simulink model "Model_1_1"  (R2024a)
settings: Solver=ode15s  StartTime=0.0  StopTime=100  FixedStep=0.0001  MaxStep=0.01  RelTol=1e-3  AbsTol=1e-3  EnableMultiTasking=on
model workspace (MATLAB code in the model file):
  | F_load_x= 2e3; %[N]
  | F_load_y= 1e4; %[N]
  | 
  | d=0.01;   %[m]
  | l=1;      %[m]
  | L=l;      %[m] Node distance
  | H=L*cos(pi/6); %[m] Node distance
  | Density=7800; %[kg/m^3]
  | E=210;   %[GPa]
  | G=79;    %[GPa]
  | bm=0.01; %[1/s] Default
  | bk=0.01; %[s] Default
  | 
  | b_rj=1; %[N*m*s/rad] Damp.Coef.Revolut joints
  | 
  | Size_frame=30; %[pixel]
undefined symbols (not defined in the file): F_x, F_y, X, Y, Z
libraries: sm_lib x58, nesl_utility x15, fl_lib x6, simulink x1
(part 1 of 2)
settings Model: NumberOfSteps=100000  Creator=Ing. Štefan Ondočko  LastModifiedBy=Ing. Štefan Ondočko
settings SolverCC: AutoScaleAbsTol=off  MaxZcPerStep=1
settings DataIOCC: LimitDataPoints=on  MaxDataPoints=10000  ReturnWorkspaceOutputs=off
settings OptimizationCC: ReuseModelBlockBuffer=off  LifeSpan=inf
settings DebuggingCC: UnconnectedInputMsg=warning  UnconnectedOutputMsg=warning  UnconnectedLineMsg=warning  AllowSymbolicDim=off  SubsystemReferenceDiagnosticForUnitTest=warning  SFUnexpectedBacktrackingDiag=warning  SFNoUnconditionalDefaultTransitionDiag=warning  SFExecutionAtInitializationDiag=none  ArithmeticOperatorsInVariantConditions=warning
settings ModelReferenceCC: EnableRefExpFcnMdlSchedulingChecks=on
settings SFSimCC: SimUseLocalCustomCode=off  CustomCodeUndefinedFunction=UseInterfaceOnly
settings RTWCC: RTWUseLocalCustomCode=off  GPUComputeCapability=3.5  DLArmComputeVersion=19.05
settings CodeAppCC: StateflowObjectComments=on
settings GRTTargetCC: TargetLangStandard=C89/C90 (ANSI)
settings ConfigComp: CovMetricSettings=dw  CovSaveCumulativeToWorkspaceVar=on  CovSaveSingleToWorkspaceVar=on  CovExternalEMLEnable=off  CovSFcnEnable=off
settings SimscapeCC: SimscapeLogType=all  SimscapeLogSimulationStatistics=on  SimscapeLogDataHistory=10000
settings ExplorerConfigSet: InternalSimMechanicsExplorerSettings="<ExplorerConfiguration><canonicalview>default</canonicalview><AnimationSetting><BasePlaybackSpeed>1.0</BasePlaybackSpeed><PlaybackSpeedFactor>2.0</PlaybackSpeedFactor></AnimationSetting><TilePanel><TileInfo><Tiles Columns=\"1\" Count=\"1\" Rows=\"1\"><Column Weight=\"1\"/><Row Weight=\"1\"/><Tile Height=\"1\" Width=\"1\" X=\"0\" Y=\"0\"/></Tiles></TileInfo><SceneInfo><SceneViewer><BGColor><R>1</R><G>1</G><B>1</B></BGColor><Camera><DoPerspective>off</DoPerspective><Position><X>1.34160017439744395</X><Y>2.43472426416735921</Y><Z>3.19868175252832421</Z></Position><Center><X>1.34160017439744395</X><Y>2.43472426416735921</Y><Z>1.1802899990698279e-08</Z></Center><Up><X>0</X><Y>1</Y><Z>-0</Z></Up><ViewLimDist>1</ViewLimDist><YLim>3.18022072065698147</YLim><XLim>1.97030216076793452</XLim></Camera></SceneViewer></SceneInfo></TilePanel><MechEditorPanel><Cameras/><GfxPanelCameraMap/><VideoCreator><PlaybackSpeedRatio>1.0</PlaybackSpeedRatio><FrameRate>30</FrameRate><VideoFormat>Motion JPEG AVI</VideoFormat><FrameSize>auto</FrameSize></VideoCreator></MechEditorPanel></ExplorerConfiguration>"

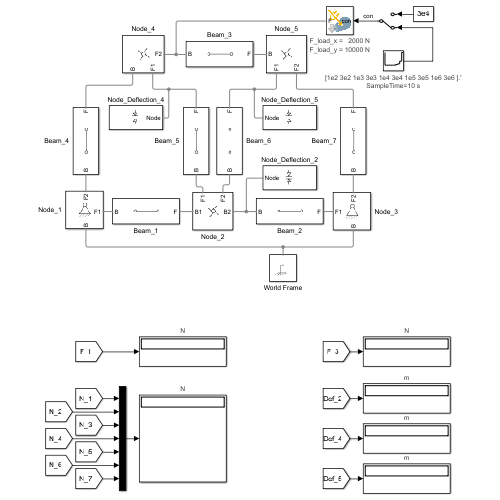
[thumbnail: Simulink's stored preview of the top-level diagram]
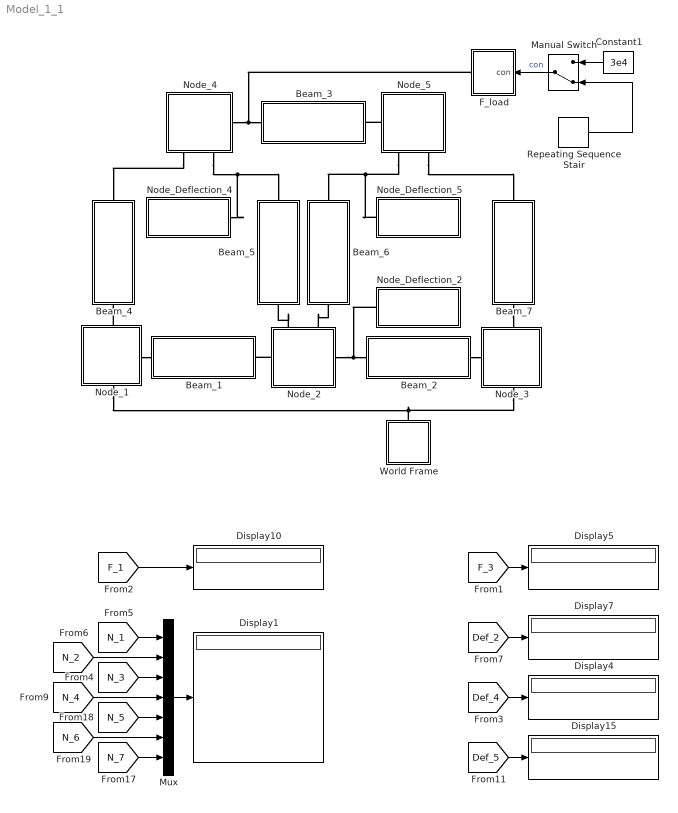
== system Model_1_1 ==
  Beam_1 : Subsystem
  Beam_2 : Subsystem
  Beam_3 : Subsystem
  Beam_4 : Subsystem
  Beam_5 : Subsystem
  Beam_6 : Subsystem
  Beam_7 : Subsystem
  Constant1 : Constant  Value=3e4
  Display{1,4..5,7,10,15} (6 alike) : Display
      Display1 settings: Description=N  AttributesFormatString=%<Description>  Format=long_e
      Display10 settings: Description=N  AttributesFormatString=%<Description>  Format=long_e
      Display15 settings: Description=m  AttributesFormatString=%<Description>  Format=long_e
      Display4 settings: Description=m  AttributesFormatString=%<Description>  Format=long_e
      Display5 settings: Description=N  AttributesFormatString=%<Description>  Format=long_e
      Display7 settings: Description=m  AttributesFormatString=%<Description>  Format=long_e
  F_load : Subsystem  mask{Fx=F_load_x, Fy=F_load_y, F=norm([F_x F_y])}
      mask prompts: Fx "Load Fx (N)"; Fy "Load Fy (N)"; F "Load F (N)"
      settings: AttributesFormatString=|
      | %<Fx> =   2000 N
      | %<Fy> = 10000 N
      mask Display: image('D:sila_F.png');
  Manual Switch : ManualSwitch  CurrentSetting=0
  Mux : Mux  Inputs=7
  Node_1 : Subsystem
      settings: PortSchema="{\"entries\":[{\"content\":{\"sides\":[{\"content\":{},\"type\":\"ConnectorPlacement.EquallySpacedRectSide\",\"uuid\":\"d437545a-b6cd-405c-92f5-dfd428dd316c\"},{\"content\":{\"connectorIds\":[\"RConn1\"],\"side\":\"RIGHT\"},\"type\":\"ConnectorPlacement.EquallySpacedRectSide\",\"uuid\":\"a6c866cb-015a-4ba6-a725-1ad5f0a48a96\"},{\"content\":{\"connectorIds\":[\"LConn1\"],\"side\":\"TOP\"},\"type\":\"ConnectorPlacement.EquallySpacedRectSide\",\"uuid\":\"8c34f49c-4b46-4dd5-857b-cc1f00e0721b\"},{\"content\":{\"connectorIds\":[\"RConn2\"],\"side\":\"BOTTOM\"},\"type\":\"ConnectorPlacement.EquallySpacedRectSide\",\"uuid\":\"e1836308-c472-4635-822e-d84e1319bcc1\"}]},\"type\":\"ConnectorPlacement.EquallySpacedConnector\",\"uuid\":\"28d0e514-5749-47ac-8c9d-469c58f8fea4\"}],\"packageUris\":[\"http://schema.mathworks.com/mf0/Connector/R2020b\"],\"version\":\"1.0\"}"
  Node_2 : Subsystem
      settings: PortSchema="{\"entries\":[{\"content\":{\"sides\":[{\"content\":{\"connectorIds\":[\"LConn1\"]},\"type\":\"ConnectorPlacement.EquallySpacedRectSide\",\"uuid\":\"afef6c51-8d1a-46bc-b1c6-0f4974bd4a7e\"},{\"content\":{\"connectorIds\":[\"RConn1\"],\"side\":\"RIGHT\"},\"type\":\"ConnectorPlacement.EquallySpacedRectSide\",\"uuid\":\"d0b349a1-0497-425d-af85-a98150ab0495\"},{\"content\":{\"side\":\"TOP\"},\"type\":\"ConnectorPlacement.EquallySpacedRectSide\",\"uuid\":\"d0ddbf7d-56c5-4c92-a64b-8a4c4ad659a6\"},{\"content\":{\"connectorIds\":[\"RConn2\",\"RConn3\"],\"side\":\"BOTTOM\"},\"type\":\"ConnectorPlacement.EquallySpacedRectSide\",\"uuid\":\"41f51937-efee-41b9-946e-3cb9cf7bb08c\"}]},\"type\":\"ConnectorPlacement.EquallySpacedConnector\",\"uuid\":\"81c85225-024f-4f40-8315-d14bb13695f6\"}],\"packageUris\":[\"http://schema.mathworks.com/mf0/Connector/R2020b\"],\"version\":\"1.0\"}"
  Node_3 : Subsystem
      settings: PortSchema="{\"entries\":[{\"content\":{\"sides\":[{\"content\":{\"connectorIds\":[\"LConn1\"]},\"type\":\"ConnectorPlacement.EquallySpacedRectSide\",\"uuid\":\"c52cac6f-2005-4bfe-89ae-e2a0406bbacd\"},{\"content\":{\"side\":\"RIGHT\"},\"type\":\"ConnectorPlacement.EquallySpacedRectSide\",\"uuid\":\"5ceadddb-1bc3-405b-9850-d33e8ff0b50d\"},{\"content\":{\"connectorIds\":[\"LConn2\"],\"side\":\"TOP\"},\"type\":\"ConnectorPlacement.EquallySpacedRectSide\",\"uuid\":\"947f3bae-c8fa-4b23-8ea1-709fee7d1677\"},{\"content\":{\"connectorIds\":[\"RConn1\"],\"side\":\"BOTTOM\"},\"type\":\"ConnectorPlacement.EquallySpacedRectSide\",\"uuid\":\"f9cd605e-29e4-49b7-a86d-9958a73b4d00\"}]},\"type\":\"ConnectorPlacement.EquallySpacedConnector\",\"uuid\":\"8856fa92-01df-438d-a79d-88950b3b721b\"}],\"packageUris\":[\"http://schema.mathworks.com/mf0/Connector/R2020b\"],\"version\":\"1.0\"}"
  Node_4 : Subsystem
      settings: PortSchema="{\"entries\":[{\"content\":{\"sides\":[{\"content\":{},\"type\":\"ConnectorPlacement.EquallySpacedRectSide\",\"uuid\":\"beaa1c3e-db26-40c7-ae29-b74306d70d13\"},{\"content\":{\"connectorIds\":[\"RConn1\"],\"side\":\"RIGHT\"},\"type\":\"ConnectorPlacement.EquallySpacedRectSide\",\"uuid\":\"a69b9587-50d9-4008-b2d1-888e5f048004\"},{\"content\":{\"connectorIds\":[\"LConn1\",\"LConn2\"],\"side\":\"TOP\"},\"type\":\"ConnectorPlacement.EquallySpacedRectSide\",\"uuid\":\"2aa7e189-65af-4eae-a330-225785720398\"}]},\"type\":\"ConnectorPlacement.EquallySpacedConnector\",\"uuid\":\"ac87f387-ad78-4612-b729-74bf7414ceb5\"}],\"packageUris\":[\"http://schema.mathworks.com/mf0/Connector/R2020b\"],\"version\":\"1.0\"}"
  Node_5 : Subsystem
      settings: PortSchema="{\"entries\":[{\"content\":{\"sides\":[{\"content\":{\"connectorIds\":[\"LConn1\"]},\"type\":\"ConnectorPlacement.EquallySpacedRectSide\",\"uuid\":\"beaa1c3e-db26-40c7-ae29-b74306d70d13\"},{\"content\":{\"side\":\"RIGHT\"},\"type\":\"ConnectorPlacement.EquallySpacedRectSide\",\"uuid\":\"a69b9587-50d9-4008-b2d1-888e5f048004\"},{\"content\":{\"connectorIds\":[\"LConn2\",\"LConn3\"],\"side\":\"TOP\"},\"type\":\"ConnectorPlacement.EquallySpacedRectSide\",\"uuid\":\"2aa7e189-65af-4eae-a330-225785720398\"}]},\"type\":\"ConnectorPlacement.EquallySpacedConnector\",\"uuid\":\"ac87f387-ad78-4612-b729-74bf7414ceb5\"}],\"packageUris\":[\"http://schema.mathworks.com/mf0/Connector/R2020b\"],\"version\":\"1.0\"}"
  Node_Deflection_2 : Subsystem
  Node_Deflection_4 : Subsystem
  Node_Deflection_5 : Subsystem
  Repeating Sequence Stair : simulink/Sources/Repeating Sequence Stair  OutValues=[1e2 3e2 1e3 3e3 1e4 3e4 1e5 3e5 1e6 3e6 ].'  tsamp=10  OutMin=[]  OutMax=[]  OutDataTypeStr=double  OutputDataTypeScalingMode=double  OutDataType=fixdt(0,8)  ConRadixGroup=Best Precision: Vector-wise  OutScaling=2^-12
      settings: AttributesFormatString=|
      | %<OutValues>
      | SampleTime=%<tsamp> s
  World Frame : Subsystem
      settings: PortSchema="{\"entries\":[{\"content\":{\"sides\":[{\"content\":{},\"type\":\"ConnectorPlacement.EquallySpacedRectSide\",\"uuid\":\"6a8e21d3-b0b2-4758-a6c8-a7be5ecb73b9\"},{\"content\":{\"side\":\"RIGHT\"},\"type\":\"ConnectorPlacement.EquallySpacedRectSide\",\"uuid\":\"42798d98-bef9-4838-9935-056c1ef1235d\"},{\"content\":{\"connectorIds\":[\"LConn1\"],\"side\":\"TOP\"},\"type\":\"ConnectorPlacement.EquallySpacedRectSide\",\"uuid\":\"7c8f84cf-9fc0-4b00-b00b-766e511bcfac\"}]},\"type\":\"ConnectorPlacement.EquallySpacedConnector\",\"uuid\":\"93a5f294-2ff9-4ffa-a830-6e6e0d522148\"}],\"packageUris\":[\"http://schema.mathworks.com/mf0/Connector/R2020b\"],\"version\":\"1.0\"}"
  wires:
  [N_1] -> Mux/1
  [F_1] -> Display10/1
  [F_3] -> Display5/1
  [Def_2] -> Display7/1
  Repeating Sequence Stair/1 -> Manual Switch/2
  Constant1/1 -> Manual Switch/1
  [Def_4] -> Display4/1
  [Def_5] -> Display15/1
  [N_2] -> Mux/2
  [N_3] -> Mux/3
  [N_4] -> Mux/4
  [N_6] -> Mux/6
  [N_5] -> Mux/5
  [N_7] -> Mux/7
  Mux/1 -> Display1/1
  Manual Switch/1 -> F_load/1(con)  "con"
  connections:
  Node_1/RConn1 -- Beam_1/LConn1
  Node_1/LConn1 -- Node_3/LConn2 -- World Frame/LConn1
  Node_1/RConn2 -- Beam_4/LConn1
  Node_2/LConn1 -- Beam_1/RConn1
  Node_2/RConn1 -- Node_Deflection_2/LConn1 -- Beam_2/LConn1
  Node_2/RConn2 -- Beam_5/LConn1
  Node_2/RConn3 -- Beam_6/LConn1
  Node_4/LConn1 -- Beam_4/RConn1
  Node_4/LConn2 -- Node_Deflection_4/LConn1 -- Beam_5/RConn1
  Node_4/RConn1 -- F_load/RConn1 -- Beam_3/LConn1
  Node_5/LConn3 -- Beam_7/RConn1
  Node_5/LConn2 -- Node_Deflection_5/LConn1 -- Beam_6/RConn1
  Node_5/LConn1 -- Beam_3/RConn1
  Beam_2/RConn1 -- Node_3/LConn1
  Beam_7/LConn1 -- Node_3/RConn1

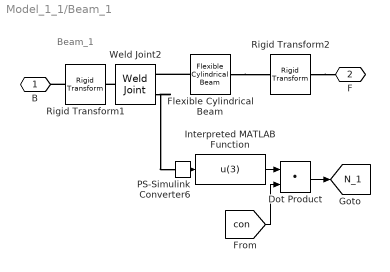
== system Model_1_1/Beam_1 ==
  note: Beam_1
  Dot Product : DotProduct  OutDataTypeStr=Inherit: Inherit via internal rule
  Flexible Cylindrical Beam : sm_lib/Body Elements/Flexible Bodies/Beams/Flexible Cylindrical Beam  SectionType=Solid  Radius=d/2  RadiusUnits=m  Thickness=1  ThicknessUnits=mm  Length=l  LengthUnits=m  StiffnessAndInertiaType=CalculateFromGeometry  Density=Density  DensityUnits=kg/m^3  ModuliType=YoungsShear  YoungsModulus=E  YoungsModulusUnits=GPa  PoissonsRatio=0.28  ShearModulus=G  ShearModulusUnits=GPa  GeometricCentroid=[0 0]  GeometricCentroidUnits=m  BendingCentroid=[0 0]  BendingCentroidUnits=m  ShearCenter=[0 0]  ShearCenterUnits=m  AxialRigidity=1  AxialRigidityUnits=Pa*m^2  FlexuralRigidity=[1 1]  FlexuralRigidityUnits=Pa*m^4  CrossFlexuralRigidity=0  CrossFlexuralRigidityUnits=Pa*m^4  TorsionalRigidity=1  TorsionalRigidityUnits=Pa*m^4  CenterOfMass=[0 0]  CenterOfMassUnits=m  MassPerUnitLength=1  MassPerUnitLengthUnits=kg/m  MassMomentOfInertiaDensity=[1 1]  MassMomentOfInertiaDensityUnits=kg*m  MassProductOfInertiaDensity=0  MassProductOfInertiaDensityUnits=kg*m  DampingType=Proportional  ProportionalDampingAlpha=bm  ProportionalDampingAlphaUnits=1/s  ProportionalDampingBeta=bk  ProportionalDampingBetaUnits=s  UniformModalDampingRatio=0.01  NumElements=1  ReductionType=None  NumRetainedModes=1  GraphicType=FromGeometry  GraphicVisPropType=SimpleVisualProperties  GraphicDiffuseColor=[0.5 0.5 0.5]  GraphicOpacity=1.0  GraphicSpecularColor=[0.5 0.5 0.5 1.0]  GraphicAmbientColor=[0.15 0.15 0.15 1.0]  GraphicEmissiveColor=[0.0 0.0 0.0 1.0]  GraphicShininess=75  DoExposeZminFrame=on  DoExposeZmaxFrame=on  SerializedFrames=<Frames/>
      settings: AttributesFormatString=%<Length>
  Interpreted MATLAB Function : MATLABFcn  Description=u(3)  MATLABFcn=u(3)
      settings: AttributesFormatString=%<Description>
  PS-Simulink Converter6 : nesl_utility/PS-Simulink Converter  PhysicalDomain=network_engine_domain  SubClassName=ps_output  LeftPortType=input  RightPortType=output  PseudoPeriodic=off  Frequencies=[]  VectorFormat=inherit  Unit=1  AffineConversion=off
  Rigid Transform1 : sm_lib/Frames and Transforms/Rigid Transform  RotationMethod=StandardAxis  FollAlignAxisA=+X  BaseAlignAxisA=+Y  FollAlignAxisB=+Y  BaseAlignAxisB=+Z  RotationStandardAxis=+Y  RotationAngle=pi/2  RotationAngleUnits=rad  RotationArbitraryAxis=[0 0 1]  RotationSequenceAxes=FollowerAxes  RotationSequence=XYX  RotationSequenceAngles=[0 0 0]  RotationSequenceAnglesUnits=deg  RotationMatrix=[1 0 0; 0 1 0; 0 0 1]  Quaternion=[1 0 0 0]  TranslationMethod=None  TranslationCartesianOffset=[0 0 0]  TranslationCartesianOffsetUnits=m  TranslationStandardAxis=+Z  TranslationStandardOffset=0  TranslationStandardOffsetUnits=m  TranslationROffset=0  TranslationROffsetUnits=m  TranslationThetaOffset=0  TranslationThetaOffsetUnits=deg  TranslationZOffset=0  TranslationZOffsetUnits=m
      settings: AttributesFormatString=|
      | %<RotationStandardAxis>
      | %<RotationAngle>
  Rigid Transform2 : sm_lib/Frames and Transforms/Rigid Transform  RotationMethod=StandardAxis  FollAlignAxisA=+X  BaseAlignAxisA=+Y  FollAlignAxisB=+Y  BaseAlignAxisB=+Z  RotationStandardAxis=+Y  RotationAngle=-pi/2  RotationAngleUnits=rad  RotationArbitraryAxis=[0 0 1]  RotationSequenceAxes=FollowerAxes  RotationSequence=XYX  RotationSequenceAngles=[0 0 0]  RotationSequenceAnglesUnits=deg  RotationMatrix=[1 0 0; 0 1 0; 0 0 1]  Quaternion=[1 0 0 0]  TranslationMethod=None  TranslationCartesianOffset=[0 0 0]  TranslationCartesianOffsetUnits=m  TranslationStandardAxis=+Z  TranslationStandardOffset=0  TranslationStandardOffsetUnits=m  TranslationROffset=0  TranslationROffsetUnits=m  TranslationThetaOffset=0  TranslationThetaOffsetUnits=deg  TranslationZOffset=0  TranslationZOffsetUnits=m
      settings: AttributesFormatString=|
      | %<RotationStandardAxis>
      | %<RotationAngle>
  Weld Joint2 : sm_lib/Joints/Weld Joint  Description=|  JointMode=Normal  CompositeWrenchDir=FollowerOnBase  CompositeWrenchFrame=BaseFrame  SenseConstraintForce=off  SenseConstraintTorque=off  SenseTotalForce=on  SenseTotalTorque=off
      | Force
      | sensing
      settings: AttributesFormatString=%<Description>
  B : PMIOPort  Side=Left
  F : PMIOPort  Port=2  Side=Right
  tag scope: N_1=global
  wires:
  PS-Simulink Converter6/1 -> Interpreted MATLAB Function/1
  [con] -> Dot Product/2
  Dot Product/1 -> [N_1]
  Interpreted MATLAB Function/1 -> Dot Product/1
  connections:
  Flexible Cylindrical Beam/LConn1 -- Weld Joint2/RConn1
  Weld Joint2/LConn1 -- Rigid Transform1/RConn1
  Rigid Transform2/RConn1 -- F/RConn1
  Flexible Cylindrical Beam/RConn1 -- Rigid Transform2/LConn1
  Rigid Transform1/LConn1 -- B/RConn1
  Weld Joint2/RConn2 -- PS-Simulink Converter6/LConn1

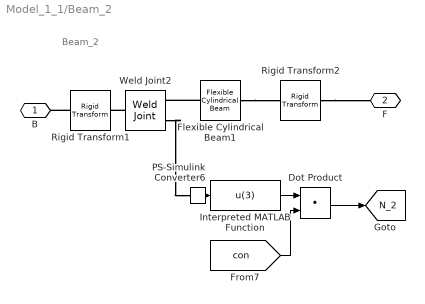
== system Model_1_1/Beam_2 ==
  note: Beam_2
  Dot Product : DotProduct  OutDataTypeStr=Inherit: Inherit via internal rule
  Flexible Cylindrical Beam1 : sm_lib/Body Elements/Flexible Bodies/Beams/Flexible Cylindrical Beam  SectionType=Solid  Radius=d/2  RadiusUnits=m  Thickness=1  ThicknessUnits=mm  Length=l  LengthUnits=m  StiffnessAndInertiaType=CalculateFromGeometry  Density=Density  DensityUnits=kg/m^3  ModuliType=YoungsShear  YoungsModulus=E  YoungsModulusUnits=GPa  PoissonsRatio=0.28  ShearModulus=G  ShearModulusUnits=GPa  GeometricCentroid=[0 0]  GeometricCentroidUnits=m  BendingCentroid=[0 0]  BendingCentroidUnits=m  ShearCenter=[0 0]  ShearCenterUnits=m  AxialRigidity=1  AxialRigidityUnits=Pa*m^2  FlexuralRigidity=[1 1]  FlexuralRigidityUnits=Pa*m^4  CrossFlexuralRigidity=0  CrossFlexuralRigidityUnits=Pa*m^4  TorsionalRigidity=1  TorsionalRigidityUnits=Pa*m^4  CenterOfMass=[0 0]  CenterOfMassUnits=m  MassPerUnitLength=1  MassPerUnitLengthUnits=kg/m  MassMomentOfInertiaDensity=[1 1]  MassMomentOfInertiaDensityUnits=kg*m  MassProductOfInertiaDensity=0  MassProductOfInertiaDensityUnits=kg*m  DampingType=Proportional  ProportionalDampingAlpha=bm  ProportionalDampingAlphaUnits=1/s  ProportionalDampingBeta=bk  ProportionalDampingBetaUnits=s  UniformModalDampingRatio=0.01  NumElements=1  ReductionType=None  NumRetainedModes=1  GraphicType=FromGeometry  GraphicVisPropType=SimpleVisualProperties  GraphicDiffuseColor=[0.5 0.5 0.5]  GraphicOpacity=1.0  GraphicSpecularColor=[0.5 0.5 0.5 1.0]  GraphicAmbientColor=[0.15 0.15 0.15 1.0]  GraphicEmissiveColor=[0.0 0.0 0.0 1.0]  GraphicShininess=75  DoExposeZminFrame=on  DoExposeZmaxFrame=on  SerializedFrames=<Frames/>
      settings: AttributesFormatString=%<Description>
  Interpreted MATLAB Function : MATLABFcn  Description=u(3)  MATLABFcn=u(3)
      settings: AttributesFormatString=%<Description>
  PS-Simulink Converter6 : nesl_utility/PS-Simulink Converter  PhysicalDomain=network_engine_domain  SubClassName=ps_output  LeftPortType=input  RightPortType=output  PseudoPeriodic=off  Frequencies=[]  VectorFormat=inherit  Unit=1  AffineConversion=off
  Rigid Transform1 : sm_lib/Frames and Transforms/Rigid Transform  RotationMethod=StandardAxis  FollAlignAxisA=+X  BaseAlignAxisA=+Y  FollAlignAxisB=+Y  BaseAlignAxisB=+Z  RotationStandardAxis=+Y  RotationAngle=90  RotationAngleUnits=deg  RotationArbitraryAxis=[0 0 1]  RotationSequenceAxes=FollowerAxes  RotationSequence=XYX  RotationSequenceAngles=[0 0 0]  RotationSequenceAnglesUnits=deg  RotationMatrix=[1 0 0; 0 1 0; 0 0 1]  Quaternion=[1 0 0 0]  TranslationMethod=None  TranslationCartesianOffset=[0 0 0]  TranslationCartesianOffsetUnits=m  TranslationStandardAxis=+Z  TranslationStandardOffset=0  TranslationStandardOffsetUnits=m  TranslationROffset=0  TranslationROffsetUnits=m  TranslationThetaOffset=0  TranslationThetaOffsetUnits=deg  TranslationZOffset=0  TranslationZOffsetUnits=m
      settings: AttributesFormatString=|
      | %<RotationStandardAxis>
      | %<RotationAngle> deg
  Rigid Transform2 : sm_lib/Frames and Transforms/Rigid Transform  RotationMethod=StandardAxis  FollAlignAxisA=+X  BaseAlignAxisA=+Y  FollAlignAxisB=+Y  BaseAlignAxisB=+Z  RotationStandardAxis=+Y  RotationAngle=-90  RotationAngleUnits=deg  RotationArbitraryAxis=[0 0 1]  RotationSequenceAxes=FollowerAxes  RotationSequence=XYX  RotationSequenceAngles=[0 0 0]  RotationSequenceAnglesUnits=deg  RotationMatrix=[1 0 0; 0 1 0; 0 0 1]  Quaternion=[1 0 0 0]  TranslationMethod=None  TranslationCartesianOffset=[0 0 0]  TranslationCartesianOffsetUnits=m  TranslationStandardAxis=+Z  TranslationStandardOffset=0  TranslationStandardOffsetUnits=m  TranslationROffset=0  TranslationROffsetUnits=m  TranslationThetaOffset=0  TranslationThetaOffsetUnits=deg  TranslationZOffset=0  TranslationZOffsetUnits=m
      settings: AttributesFormatString=|
      | %<RotationStandardAxis>
      | %<RotationAngle> deg
  Weld Joint2 : sm_lib/Joints/Weld Joint  Description=|  JointMode=Normal  CompositeWrenchDir=FollowerOnBase  CompositeWrenchFrame=BaseFrame  SenseConstraintForce=off  SenseConstraintTorque=off  SenseTotalForce=on  SenseTotalTorque=off
      | Total force
      | sensing
      settings: AttributesFormatString=%<Description>
  B : PMIOPort  Side=Left
  F : PMIOPort  Port=2  Side=Right
  tag scope: N_2=global
  wires:
  Dot Product/1 -> [N_2]
  [con] -> Dot Product/2
  Interpreted MATLAB Function/1 -> Dot Product/1
  PS-Simulink Converter6/1 -> Interpreted MATLAB Function/1
  connections:
  Weld Joint2/RConn2 -- PS-Simulink Converter6/LConn1
  Rigid Transform1/LConn1 -- B/RConn1
  Flexible Cylindrical Beam1/RConn1 -- Rigid Transform2/LConn1
  Rigid Transform2/RConn1 -- F/RConn1
  Weld Joint2/LConn1 -- Rigid Transform1/RConn1
  Flexible Cylindrical Beam1/LConn1 -- Weld Joint2/RConn1

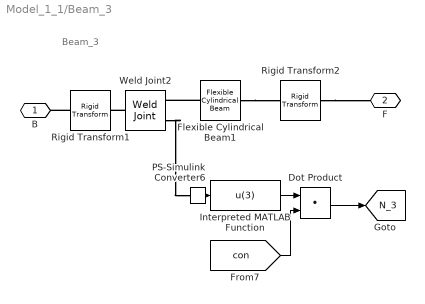
== system Model_1_1/Beam_3 ==
  note: Beam_3
  Dot Product : DotProduct  OutDataTypeStr=Inherit: Inherit via internal rule
  Flexible Cylindrical Beam1 : sm_lib/Body Elements/Flexible Bodies/Beams/Flexible Cylindrical Beam  SectionType=Solid  Radius=d/2  RadiusUnits=m  Thickness=1  ThicknessUnits=mm  Length=l  LengthUnits=m  StiffnessAndInertiaType=CalculateFromGeometry  Density=Density  DensityUnits=kg/m^3  ModuliType=YoungsShear  YoungsModulus=E  YoungsModulusUnits=GPa  PoissonsRatio=0.28  ShearModulus=G  ShearModulusUnits=GPa  GeometricCentroid=[0 0]  GeometricCentroidUnits=m  BendingCentroid=[0 0]  BendingCentroidUnits=m  ShearCenter=[0 0]  ShearCenterUnits=m  AxialRigidity=1  AxialRigidityUnits=Pa*m^2  FlexuralRigidity=[1 1]  FlexuralRigidityUnits=Pa*m^4  CrossFlexuralRigidity=0  CrossFlexuralRigidityUnits=Pa*m^4  TorsionalRigidity=1  TorsionalRigidityUnits=Pa*m^4  CenterOfMass=[0 0]  CenterOfMassUnits=m  MassPerUnitLength=1  MassPerUnitLengthUnits=kg/m  MassMomentOfInertiaDensity=[1 1]  MassMomentOfInertiaDensityUnits=kg*m  MassProductOfInertiaDensity=0  MassProductOfInertiaDensityUnits=kg*m  DampingType=Proportional  ProportionalDampingAlpha=bm  ProportionalDampingAlphaUnits=1/s  ProportionalDampingBeta=bk  ProportionalDampingBetaUnits=s  UniformModalDampingRatio=0.01  NumElements=1  ReductionType=None  NumRetainedModes=1  GraphicType=FromGeometry  GraphicVisPropType=SimpleVisualProperties  GraphicDiffuseColor=[0.5 0.5 0.5]  GraphicOpacity=1.0  GraphicSpecularColor=[0.5 0.5 0.5 1.0]  GraphicAmbientColor=[0.15 0.15 0.15 1.0]  GraphicEmissiveColor=[0.0 0.0 0.0 1.0]  GraphicShininess=75  DoExposeZminFrame=on  DoExposeZmaxFrame=on  SerializedFrames=<Frames/>
      settings: AttributesFormatString=%<Description>
  Interpreted MATLAB Function : MATLABFcn  Description=u(3)  MATLABFcn=u(3)
      settings: AttributesFormatString=%<Description>
  PS-Simulink Converter6 : nesl_utility/PS-Simulink Converter  PhysicalDomain=network_engine_domain  SubClassName=ps_output  LeftPortType=input  RightPortType=output  PseudoPeriodic=off  Frequencies=[]  VectorFormat=inherit  Unit=1  AffineConversion=off
  Rigid Transform1 : sm_lib/Frames and Transforms/Rigid Transform  RotationMethod=StandardAxis  FollAlignAxisA=+X  BaseAlignAxisA=+Y  FollAlignAxisB=+Y  BaseAlignAxisB=+Z  RotationStandardAxis=+Y  RotationAngle=90  RotationAngleUnits=deg  RotationArbitraryAxis=[0 0 1]  RotationSequenceAxes=FollowerAxes  RotationSequence=XYX  RotationSequenceAngles=[0 0 0]  RotationSequenceAnglesUnits=deg  RotationMatrix=[1 0 0; 0 1 0; 0 0 1]  Quaternion=[1 0 0 0]  TranslationMethod=None  TranslationCartesianOffset=[0 0 0]  TranslationCartesianOffsetUnits=m  TranslationStandardAxis=+Z  TranslationStandardOffset=0  TranslationStandardOffsetUnits=m  TranslationROffset=0  TranslationROffsetUnits=m  TranslationThetaOffset=0  TranslationThetaOffsetUnits=deg  TranslationZOffset=0  TranslationZOffsetUnits=m
      settings: AttributesFormatString=|
      | %<RotationStandardAxis>
      | %<RotationAngle> deg
  Rigid Transform2 : sm_lib/Frames and Transforms/Rigid Transform  RotationMethod=StandardAxis  FollAlignAxisA=+X  BaseAlignAxisA=+Y  FollAlignAxisB=+Y  BaseAlignAxisB=+Z  RotationStandardAxis=+Y  RotationAngle=-90  RotationAngleUnits=deg  RotationArbitraryAxis=[0 0 1]  RotationSequenceAxes=FollowerAxes  RotationSequence=XYX  RotationSequenceAngles=[0 0 0]  RotationSequenceAnglesUnits=deg  RotationMatrix=[1 0 0; 0 1 0; 0 0 1]  Quaternion=[1 0 0 0]  TranslationMethod=None  TranslationCartesianOffset=[0 0 0]  TranslationCartesianOffsetUnits=m  TranslationStandardAxis=+Z  TranslationStandardOffset=0  TranslationStandardOffsetUnits=m  TranslationROffset=0  TranslationROffsetUnits=m  TranslationThetaOffset=0  TranslationThetaOffsetUnits=deg  TranslationZOffset=0  TranslationZOffsetUnits=m
      settings: AttributesFormatString=|
      | %<RotationStandardAxis>
      | %<RotationAngle> deg
  Weld Joint2 : sm_lib/Joints/Weld Joint  Description=|  JointMode=Normal  CompositeWrenchDir=FollowerOnBase  CompositeWrenchFrame=BaseFrame  SenseConstraintForce=off  SenseConstraintTorque=off  SenseTotalForce=on  SenseTotalTorque=off
      | Total force
      | sensing
      settings: AttributesFormatString=%<Description>
  B : PMIOPort  Side=Left
  F : PMIOPort  Port=2  Side=Right
  tag scope: N_3=global
  wires:
  Dot Product/1 -> [N_3]
  [con] -> Dot Product/2
  Interpreted MATLAB Function/1 -> Dot Product/1
  PS-Simulink Converter6/1 -> Interpreted MATLAB Function/1
  connections:
  Weld Joint2/RConn2 -- PS-Simulink Converter6/LConn1
  Rigid Transform1/LConn1 -- B/RConn1
  Flexible Cylindrical Beam1/RConn1 -- Rigid Transform2/LConn1
  Rigid Transform2/RConn1 -- F/RConn1
  Weld Joint2/LConn1 -- Rigid Transform1/RConn1
  Flexible Cylindrical Beam1/LConn1 -- Weld Joint2/RConn1

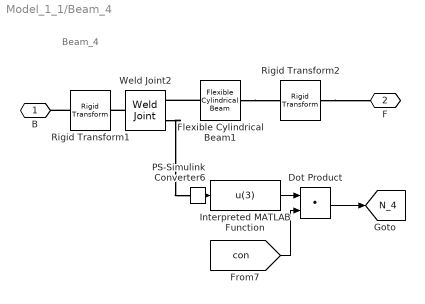
== system Model_1_1/Beam_4 ==
  note: Beam_4
  Dot Product : DotProduct  OutDataTypeStr=Inherit: Inherit via internal rule
  Flexible Cylindrical Beam1 : sm_lib/Body Elements/Flexible Bodies/Beams/Flexible Cylindrical Beam  SectionType=Solid  Radius=d/2  RadiusUnits=m  Thickness=1  ThicknessUnits=mm  Length=l  LengthUnits=m  StiffnessAndInertiaType=CalculateFromGeometry  Density=Density  DensityUnits=kg/m^3  ModuliType=YoungsShear  YoungsModulus=E  YoungsModulusUnits=GPa  PoissonsRatio=0.28  ShearModulus=G  ShearModulusUnits=GPa  GeometricCentroid=[0 0]  GeometricCentroidUnits=m  BendingCentroid=[0 0]  BendingCentroidUnits=m  ShearCenter=[0 0]  ShearCenterUnits=m  AxialRigidity=1  AxialRigidityUnits=Pa*m^2  FlexuralRigidity=[1 1]  FlexuralRigidityUnits=Pa*m^4  CrossFlexuralRigidity=0  CrossFlexuralRigidityUnits=Pa*m^4  TorsionalRigidity=1  TorsionalRigidityUnits=Pa*m^4  CenterOfMass=[0 0]  CenterOfMassUnits=m  MassPerUnitLength=1  MassPerUnitLengthUnits=kg/m  MassMomentOfInertiaDensity=[1 1]  MassMomentOfInertiaDensityUnits=kg*m  MassProductOfInertiaDensity=0  MassProductOfInertiaDensityUnits=kg*m  DampingType=Proportional  ProportionalDampingAlpha=bm  ProportionalDampingAlphaUnits=1/s  ProportionalDampingBeta=bk  ProportionalDampingBetaUnits=s  UniformModalDampingRatio=0.01  NumElements=1  ReductionType=None  NumRetainedModes=1  GraphicType=FromGeometry  GraphicVisPropType=SimpleVisualProperties  GraphicDiffuseColor=[0.5 0.5 0.5]  GraphicOpacity=1.0  GraphicSpecularColor=[0.5 0.5 0.5 1.0]  GraphicAmbientColor=[0.15 0.15 0.15 1.0]  GraphicEmissiveColor=[0.0 0.0 0.0 1.0]  GraphicShininess=75  DoExposeZminFrame=on  DoExposeZmaxFrame=on  SerializedFrames=<Frames/>
      settings: AttributesFormatString=%<Description>
  Interpreted MATLAB Function : MATLABFcn  Description=u(3)  MATLABFcn=u(3)
      settings: AttributesFormatString=%<Description>
  PS-Simulink Converter6 : nesl_utility/PS-Simulink Converter  PhysicalDomain=network_engine_domain  SubClassName=ps_output  LeftPortType=input  RightPortType=output  PseudoPeriodic=off  Frequencies=[]  VectorFormat=inherit  Unit=1  AffineConversion=off
  Rigid Transform1 : sm_lib/Frames and Transforms/Rigid Transform  RotationMethod=StandardAxis  FollAlignAxisA=+X  BaseAlignAxisA=+Y  FollAlignAxisB=+Y  BaseAlignAxisB=+Z  RotationStandardAxis=+Y  RotationAngle=90  RotationAngleUnits=deg  RotationArbitraryAxis=[0 0 1]  RotationSequenceAxes=FollowerAxes  RotationSequence=XYX  RotationSequenceAngles=[0 0 0]  RotationSequenceAnglesUnits=deg  RotationMatrix=[1 0 0; 0 1 0; 0 0 1]  Quaternion=[1 0 0 0]  TranslationMethod=None  TranslationCartesianOffset=[0 0 0]  TranslationCartesianOffsetUnits=m  TranslationStandardAxis=+Z  TranslationStandardOffset=0  TranslationStandardOffsetUnits=m  TranslationROffset=0  TranslationROffsetUnits=m  TranslationThetaOffset=0  TranslationThetaOffsetUnits=deg  TranslationZOffset=0  TranslationZOffsetUnits=m
      settings: AttributesFormatString=|
      | %<RotationStandardAxis>
      | %<RotationAngle> deg
  Rigid Transform2 : sm_lib/Frames and Transforms/Rigid Transform  RotationMethod=StandardAxis  FollAlignAxisA=+X  BaseAlignAxisA=+Y  FollAlignAxisB=+Y  BaseAlignAxisB=+Z  RotationStandardAxis=+Y  RotationAngle=-90  RotationAngleUnits=deg  RotationArbitraryAxis=[0 0 1]  RotationSequenceAxes=FollowerAxes  RotationSequence=XYX  RotationSequenceAngles=[0 0 0]  RotationSequenceAnglesUnits=deg  RotationMatrix=[1 0 0; 0 1 0; 0 0 1]  Quaternion=[1 0 0 0]  TranslationMethod=None  TranslationCartesianOffset=[0 0 0]  TranslationCartesianOffsetUnits=m  TranslationStandardAxis=+Z  TranslationStandardOffset=0  TranslationStandardOffsetUnits=m  TranslationROffset=0  TranslationROffsetUnits=m  TranslationThetaOffset=0  TranslationThetaOffsetUnits=deg  TranslationZOffset=0  TranslationZOffsetUnits=m
      settings: AttributesFormatString=|
      | %<RotationStandardAxis>
      | %<RotationAngle> deg
  Weld Joint2 : sm_lib/Joints/Weld Joint  Description=|  JointMode=Normal  CompositeWrenchDir=FollowerOnBase  CompositeWrenchFrame=BaseFrame  SenseConstraintForce=off  SenseConstraintTorque=off  SenseTotalForce=on  SenseTotalTorque=off
      | Total force
      | sensing
      settings: AttributesFormatString=%<Description>
  B : PMIOPort  Side=Left
  F : PMIOPort  Port=2  Side=Right
  tag scope: N_4=global
  wires:
  Interpreted MATLAB Function/1 -> Dot Product/1
  Dot Product/1 -> [N_4]
  PS-Simulink Converter6/1 -> Interpreted MATLAB Function/1
  [con] -> Dot Product/2
  connections:
  Weld Joint2/LConn1 -- Rigid Transform1/RConn1
  Flexible Cylindrical Beam1/LConn1 -- Weld Joint2/RConn1
  Rigid Transform1/LConn1 -- B/RConn1
  Rigid Transform2/RConn1 -- F/RConn1
  Flexible Cylindrical Beam1/RConn1 -- Rigid Transform2/LConn1
  Weld Joint2/RConn2 -- PS-Simulink Converter6/LConn1

== system Model_1_1/Beam_5 ==
  note: Beam_5
  Dot Product : DotProduct  OutDataTypeStr=Inherit: Inherit via internal rule
  Flexible Cylindrical Beam1 : sm_lib/Body Elements/Flexible Bodies/Beams/Flexible Cylindrical Beam  SectionType=Solid  Radius=d/2  RadiusUnits=m  Thickness=1  ThicknessUnits=mm  Length=l  LengthUnits=m  StiffnessAndInertiaType=CalculateFromGeometry  Density=Density  DensityUnits=kg/m^3  ModuliType=YoungsShear  YoungsModulus=E  YoungsModulusUnits=GPa  PoissonsRatio=0.28  ShearModulus=G  ShearModulusUnits=GPa  GeometricCentroid=[0 0]  GeometricCentroidUnits=m  BendingCentroid=[0 0]  BendingCentroidUnits=m  ShearCenter=[0 0]  ShearCenterUnits=m  AxialRigidity=1  AxialRigidityUnits=Pa*m^2  FlexuralRigidity=[1 1]  FlexuralRigidityUnits=Pa*m^4  CrossFlexuralRigidity=0  CrossFlexuralRigidityUnits=Pa*m^4  TorsionalRigidity=1  TorsionalRigidityUnits=Pa*m^4  CenterOfMass=[0 0]  CenterOfMassUnits=m  MassPerUnitLength=1  MassPerUnitLengthUnits=kg/m  MassMomentOfInertiaDensity=[1 1]  MassMomentOfInertiaDensityUnits=kg*m  MassProductOfInertiaDensity=0  MassProductOfInertiaDensityUnits=kg*m  DampingType=Proportional  ProportionalDampingAlpha=bm  ProportionalDampingAlphaUnits=1/s  ProportionalDampingBeta=bk  ProportionalDampingBetaUnits=s  UniformModalDampingRatio=0.01  NumElements=1  ReductionType=None  NumRetainedModes=1  GraphicType=FromGeometry  GraphicVisPropType=SimpleVisualProperties  GraphicDiffuseColor=[0.5 0.5 0.5]  GraphicOpacity=1.0  GraphicSpecularColor=[0.5 0.5 0.5 1.0]  GraphicAmbientColor=[0.15 0.15 0.15 1.0]  GraphicEmissiveColor=[0.0 0.0 0.0 1.0]  GraphicShininess=75  DoExposeZminFrame=on  DoExposeZmaxFrame=on  SerializedFrames=<Frames/>
      settings: AttributesFormatString=%<Description>
  Interpreted MATLAB Function : MATLABFcn  Description=u(3)  MATLABFcn=u(3)
      settings: AttributesFormatString=%<Description>
  PS-Simulink Converter6 : nesl_utility/PS-Simulink Converter  PhysicalDomain=network_engine_domain  SubClassName=ps_output  LeftPortType=input  RightPortType=output  PseudoPeriodic=off  Frequencies=[]  VectorFormat=inherit  Unit=1  AffineConversion=off
  Rigid Transform1 : sm_lib/Frames and Transforms/Rigid Transform  RotationMethod=StandardAxis  FollAlignAxisA=+X  BaseAlignAxisA=+Y  FollAlignAxisB=+Y  BaseAlignAxisB=+Z  RotationStandardAxis=+Y  RotationAngle=90  RotationAngleUnits=deg  RotationArbitraryAxis=[0 0 1]  RotationSequenceAxes=FollowerAxes  RotationSequence=XYX  RotationSequenceAngles=[0 0 0]  RotationSequenceAnglesUnits=deg  RotationMatrix=[1 0 0; 0 1 0; 0 0 1]  Quaternion=[1 0 0 0]  TranslationMethod=None  TranslationCartesianOffset=[0 0 0]  TranslationCartesianOffsetUnits=m  TranslationStandardAxis=+Z  TranslationStandardOffset=0  TranslationStandardOffsetUnits=m  TranslationROffset=0  TranslationROffsetUnits=m  TranslationThetaOffset=0  TranslationThetaOffsetUnits=deg  TranslationZOffset=0  TranslationZOffsetUnits=m
      settings: AttributesFormatString=|
      | %<RotationStandardAxis>
      | %<RotationAngle> deg
  Rigid Transform2 : sm_lib/Frames and Transforms/Rigid Transform  RotationMethod=StandardAxis  FollAlignAxisA=+X  BaseAlignAxisA=+Y  FollAlignAxisB=+Y  BaseAlignAxisB=+Z  RotationStandardAxis=+Y  RotationAngle=-90  RotationAngleUnits=deg  RotationArbitraryAxis=[0 0 1]  RotationSequenceAxes=FollowerAxes  RotationSequence=XYX  RotationSequenceAngles=[0 0 0]  RotationSequenceAnglesUnits=deg  RotationMatrix=[1 0 0; 0 1 0; 0 0 1]  Quaternion=[1 0 0 0]  TranslationMethod=None  TranslationCartesianOffset=[0 0 0]  TranslationCartesianOffsetUnits=m  TranslationStandardAxis=+Z  TranslationStandardOffset=0  TranslationStandardOffsetUnits=m  TranslationROffset=0  TranslationROffsetUnits=m  TranslationThetaOffset=0  TranslationThetaOffsetUnits=deg  TranslationZOffset=0  TranslationZOffsetUnits=m
      settings: AttributesFormatString=|
      | %<RotationStandardAxis>
      | %<RotationAngle> deg
  Weld Joint2 : sm_lib/Joints/Weld Joint  Description=|  JointMode=Normal  CompositeWrenchDir=FollowerOnBase  CompositeWrenchFrame=BaseFrame  SenseConstraintForce=off  SenseConstraintTorque=off  SenseTotalForce=on  SenseTotalTorque=off
      | Total force
      | sensing
      settings: AttributesFormatString=%<Description>
  B : PMIOPort  Side=Left
  F : PMIOPort  Port=2  Side=Right
  tag scope: N_5=global
  wires:
  [con] -> Dot Product/2
  PS-Simulink Converter6/1 -> Interpreted MATLAB Function/1
  Dot Product/1 -> [N_5]
  Interpreted MATLAB Function/1 -> Dot Product/1
  connections:
  Weld Joint2/RConn2 -- PS-Simulink Converter6/LConn1
  Flexible Cylindrical Beam1/RConn1 -- Rigid Transform2/LConn1
  Rigid Transform2/RConn1 -- F/RConn1
  Rigid Transform1/LConn1 -- B/RConn1
  Flexible Cylindrical Beam1/LConn1 -- Weld Joint2/RConn1
  Weld Joint2/LConn1 -- Rigid Transform1/RConn1

== system Model_1_1/Beam_6 ==
  note: Beam_6
  Dot Product : DotProduct  OutDataTypeStr=Inherit: Inherit via internal rule
  Flexible Cylindrical Beam1 : sm_lib/Body Elements/Flexible Bodies/Beams/Flexible Cylindrical Beam  SectionType=Solid  Radius=d/2  RadiusUnits=m  Thickness=1  ThicknessUnits=mm  Length=l  LengthUnits=m  StiffnessAndInertiaType=CalculateFromGeometry  Density=Density  DensityUnits=kg/m^3  ModuliType=YoungsShear  YoungsModulus=E  YoungsModulusUnits=GPa  PoissonsRatio=0.28  ShearModulus=G  ShearModulusUnits=GPa  GeometricCentroid=[0 0]  GeometricCentroidUnits=m  BendingCentroid=[0 0]  BendingCentroidUnits=m  ShearCenter=[0 0]  ShearCenterUnits=m  AxialRigidity=1  AxialRigidityUnits=Pa*m^2  FlexuralRigidity=[1 1]  FlexuralRigidityUnits=Pa*m^4  CrossFlexuralRigidity=0  CrossFlexuralRigidityUnits=Pa*m^4  TorsionalRigidity=1  TorsionalRigidityUnits=Pa*m^4  CenterOfMass=[0 0]  CenterOfMassUnits=m  MassPerUnitLength=1  MassPerUnitLengthUnits=kg/m  MassMomentOfInertiaDensity=[1 1]  MassMomentOfInertiaDensityUnits=kg*m  MassProductOfInertiaDensity=0  MassProductOfInertiaDensityUnits=kg*m  DampingType=Proportional  ProportionalDampingAlpha=bm  ProportionalDampingAlphaUnits=1/s  ProportionalDampingBeta=bk  ProportionalDampingBetaUnits=s  UniformModalDampingRatio=0.01  NumElements=1  ReductionType=None  NumRetainedModes=1  GraphicType=FromGeometry  GraphicVisPropType=SimpleVisualProperties  GraphicDiffuseColor=[0.5 0.5 0.5]  GraphicOpacity=1.0  GraphicSpecularColor=[0.5 0.5 0.5 1.0]  GraphicAmbientColor=[0.15 0.15 0.15 1.0]  GraphicEmissiveColor=[0.0 0.0 0.0 1.0]  GraphicShininess=75  DoExposeZminFrame=on  DoExposeZmaxFrame=on  SerializedFrames=<Frames/>
      settings: AttributesFormatString=%<Description>
  Interpreted MATLAB Function : MATLABFcn  Description=u(3)  MATLABFcn=u(3)
      settings: AttributesFormatString=%<Description>
  PS-Simulink Converter6 : nesl_utility/PS-Simulink Converter  PhysicalDomain=network_engine_domain  SubClassName=ps_output  LeftPortType=input  RightPortType=output  PseudoPeriodic=off  Frequencies=[]  VectorFormat=inherit  Unit=1  AffineConversion=off
  Rigid Transform1 : sm_lib/Frames and Transforms/Rigid Transform  RotationMethod=StandardAxis  FollAlignAxisA=+X  BaseAlignAxisA=+Y  FollAlignAxisB=+Y  BaseAlignAxisB=+Z  RotationStandardAxis=+Y  RotationAngle=90  RotationAngleUnits=deg  RotationArbitraryAxis=[0 0 1]  RotationSequenceAxes=FollowerAxes  RotationSequence=XYX  RotationSequenceAngles=[0 0 0]  RotationSequenceAnglesUnits=deg  RotationMatrix=[1 0 0; 0 1 0; 0 0 1]  Quaternion=[1 0 0 0]  TranslationMethod=None  TranslationCartesianOffset=[0 0 0]  TranslationCartesianOffsetUnits=m  TranslationStandardAxis=+Z  TranslationStandardOffset=0  TranslationStandardOffsetUnits=m  TranslationROffset=0  TranslationROffsetUnits=m  TranslationThetaOffset=0  TranslationThetaOffsetUnits=deg  TranslationZOffset=0  TranslationZOffsetUnits=m
      settings: AttributesFormatString=|
      | %<RotationStandardAxis>
      | %<RotationAngle> deg
  Rigid Transform2 : sm_lib/Frames and Transforms/Rigid Transform  RotationMethod=StandardAxis  FollAlignAxisA=+X  BaseAlignAxisA=+Y  FollAlignAxisB=+Y  BaseAlignAxisB=+Z  RotationStandardAxis=+Y  RotationAngle=-90  RotationAngleUnits=deg  RotationArbitraryAxis=[0 0 1]  RotationSequenceAxes=FollowerAxes  RotationSequence=XYX  RotationSequenceAngles=[0 0 0]  RotationSequenceAnglesUnits=deg  RotationMatrix=[1 0 0; 0 1 0; 0 0 1]  Quaternion=[1 0 0 0]  TranslationMethod=None  TranslationCartesianOffset=[0 0 0]  TranslationCartesianOffsetUnits=m  TranslationStandardAxis=+Z  TranslationStandardOffset=0  TranslationStandardOffsetUnits=m  TranslationROffset=0  TranslationROffsetUnits=m  TranslationThetaOffset=0  TranslationThetaOffsetUnits=deg  TranslationZOffset=0  TranslationZOffsetUnits=m
      settings: AttributesFormatString=|
      | %<RotationStandardAxis>
      | %<RotationAngle> deg
  Weld Joint2 : sm_lib/Joints/Weld Joint  Description=|  JointMode=Normal  CompositeWrenchDir=FollowerOnBase  CompositeWrenchFrame=BaseFrame  SenseConstraintForce=off  SenseConstraintTorque=off  SenseTotalForce=on  SenseTotalTorque=off
      | Total force
      | sensing
      settings: AttributesFormatString=%<Description>
  B : PMIOPort  Side=Left
  F : PMIOPort  Port=2  Side=Right
  tag scope: N_6=global
  wires:
  Interpreted MATLAB Function/1 -> Dot Product/1
  Dot Product/1 -> [N_6]
  PS-Simulink Converter6/1 -> Interpreted MATLAB Function/1
  [con] -> Dot Product/2
  connections:
  Weld Joint2/LConn1 -- Rigid Transform1/RConn1
  Flexible Cylindrical Beam1/LConn1 -- Weld Joint2/RConn1
  Rigid Transform1/LConn1 -- B/RConn1
  Rigid Transform2/RConn1 -- F/RConn1
  Flexible Cylindrical Beam1/RConn1 -- Rigid Transform2/LConn1
  Weld Joint2/RConn2 -- PS-Simulink Converter6/LConn1

== system Model_1_1/Beam_7 ==
  note: Beam_7
  Dot Product : DotProduct  OutDataTypeStr=Inherit: Inherit via internal rule
  Flexible Cylindrical Beam1 : sm_lib/Body Elements/Flexible Bodies/Beams/Flexible Cylindrical Beam  SectionType=Solid  Radius=d/2  RadiusUnits=m  Thickness=1  ThicknessUnits=mm  Length=l  LengthUnits=m  StiffnessAndInertiaType=CalculateFromGeometry  Density=Density  DensityUnits=kg/m^3  ModuliType=YoungsShear  YoungsModulus=E  YoungsModulusUnits=GPa  PoissonsRatio=0.28  ShearModulus=G  ShearModulusUnits=GPa  GeometricCentroid=[0 0]  GeometricCentroidUnits=m  BendingCentroid=[0 0]  BendingCentroidUnits=m  ShearCenter=[0 0]  ShearCenterUnits=m  AxialRigidity=1  AxialRigidityUnits=Pa*m^2  FlexuralRigidity=[1 1]  FlexuralRigidityUnits=Pa*m^4  CrossFlexuralRigidity=0  CrossFlexuralRigidityUnits=Pa*m^4  TorsionalRigidity=1  TorsionalRigidityUnits=Pa*m^4  CenterOfMass=[0 0]  CenterOfMassUnits=m  MassPerUnitLength=1  MassPerUnitLengthUnits=kg/m  MassMomentOfInertiaDensity=[1 1]  MassMomentOfInertiaDensityUnits=kg*m  MassProductOfInertiaDensity=0  MassProductOfInertiaDensityUnits=kg*m  DampingType=Proportional  ProportionalDampingAlpha=bm  ProportionalDampingAlphaUnits=1/s  ProportionalDampingBeta=bk  ProportionalDampingBetaUnits=s  UniformModalDampingRatio=0.01  NumElements=1  ReductionType=None  NumRetainedModes=1  GraphicType=FromGeometry  GraphicVisPropType=SimpleVisualProperties  GraphicDiffuseColor=[0.5 0.5 0.5]  GraphicOpacity=1.0  GraphicSpecularColor=[0.5 0.5 0.5 1.0]  GraphicAmbientColor=[0.15 0.15 0.15 1.0]  GraphicEmissiveColor=[0.0 0.0 0.0 1.0]  GraphicShininess=75  DoExposeZminFrame=on  DoExposeZmaxFrame=on  SerializedFrames=<Frames/>
      settings: AttributesFormatString=%<Description>
  Interpreted MATLAB Function : MATLABFcn  Description=u(3)  MATLABFcn=u(3)
      settings: AttributesFormatString=%<Description>
  PS-Simulink Converter6 : nesl_utility/PS-Simulink Converter  PhysicalDomain=network_engine_domain  SubClassName=ps_output  LeftPortType=input  RightPortType=output  PseudoPeriodic=off  Frequencies=[]  VectorFormat=inherit  Unit=1  AffineConversion=off
  Rigid Transform1 : sm_lib/Frames and Transforms/Rigid Transform  RotationMethod=StandardAxis  FollAlignAxisA=+X  BaseAlignAxisA=+Y  FollAlignAxisB=+Y  BaseAlignAxisB=+Z  RotationStandardAxis=+Y  RotationAngle=90  RotationAngleUnits=deg  RotationArbitraryAxis=[0 0 1]  RotationSequenceAxes=FollowerAxes  RotationSequence=XYX  RotationSequenceAngles=[0 0 0]  RotationSequenceAnglesUnits=deg  RotationMatrix=[1 0 0; 0 1 0; 0 0 1]  Quaternion=[1 0 0 0]  TranslationMethod=None  TranslationCartesianOffset=[0 0 0]  TranslationCartesianOffsetUnits=m  TranslationStandardAxis=+Z  TranslationStandardOffset=0  TranslationStandardOffsetUnits=m  TranslationROffset=0  TranslationROffsetUnits=m  TranslationThetaOffset=0  TranslationThetaOffsetUnits=deg  TranslationZOffset=0  TranslationZOffsetUnits=m
      settings: AttributesFormatString=|
      | %<RotationStandardAxis>
      | %<RotationAngle> deg
  Rigid Transform2 : sm_lib/Frames and Transforms/Rigid Transform  RotationMethod=StandardAxis  FollAlignAxisA=+X  BaseAlignAxisA=+Y  FollAlignAxisB=+Y  BaseAlignAxisB=+Z  RotationStandardAxis=+Y  RotationAngle=-90  RotationAngleUnits=deg  RotationArbitraryAxis=[0 0 1]  RotationSequenceAxes=FollowerAxes  RotationSequence=XYX  RotationSequenceAngles=[0 0 0]  RotationSequenceAnglesUnits=deg  RotationMatrix=[1 0 0; 0 1 0; 0 0 1]  Quaternion=[1 0 0 0]  TranslationMethod=None  TranslationCartesianOffset=[0 0 0]  TranslationCartesianOffsetUnits=m  TranslationStandardAxis=+Z  TranslationStandardOffset=0  TranslationStandardOffsetUnits=m  TranslationROffset=0  TranslationROffsetUnits=m  TranslationThetaOffset=0  TranslationThetaOffsetUnits=deg  TranslationZOffset=0  TranslationZOffsetUnits=m
      settings: AttributesFormatString=|
      | %<RotationStandardAxis>
      | %<RotationAngle> deg
  Weld Joint2 : sm_lib/Joints/Weld Joint  Description=|  JointMode=Normal  CompositeWrenchDir=FollowerOnBase  CompositeWrenchFrame=BaseFrame  SenseConstraintForce=off  SenseConstraintTorque=off  SenseTotalForce=on  SenseTotalTorque=off
      | Total force
      | sensing
      settings: AttributesFormatString=%<Description>
  B : PMIOPort  Side=Left
  F : PMIOPort  Port=2  Side=Right
  tag scope: N_7=global
  wires:
  [con] -> Dot Product/2
  PS-Simulink Converter6/1 -> Interpreted MATLAB Function/1
  Dot Product/1 -> [N_7]
  Interpreted MATLAB Function/1 -> Dot Product/1
  connections:
  Weld Joint2/RConn2 -- PS-Simulink Converter6/LConn1
  Flexible Cylindrical Beam1/RConn1 -- Rigid Transform2/LConn1
  Rigid Transform2/RConn1 -- F/RConn1
  Rigid Transform1/LConn1 -- B/RConn1
  Flexible Cylindrical Beam1/LConn1 -- Weld Joint2/RConn1
  Weld Joint2/LConn1 -- Rigid Transform1/RConn1

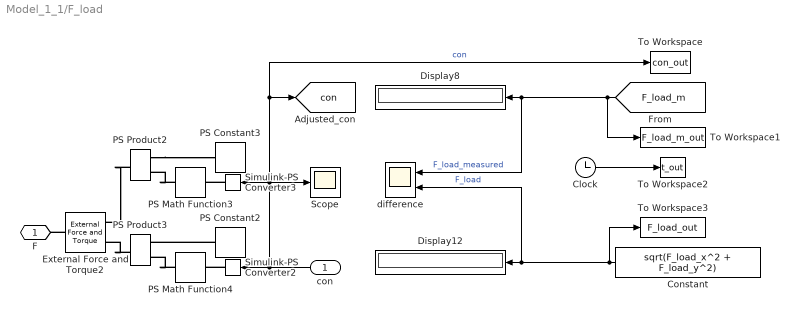
== system Model_1_1/F_load ==
  con : Inport
  Clock : Clock
  Constant : Constant  Value=sqrt(F_load_x^2 + F_load_y^2)
  Display12 : Display
      settings: Description=N  AttributesFormatString=%<Description>  Format=long_e
  Display8 : Display
      settings: Description=N  AttributesFormatString=%<Description>  Format=long_e
  External Force and Torque2 : sm_lib/Forces and Torques/External Force and Torque  EnableForceX=on  EnableForceY=on  EnableForceZ=off  EnableForce=off  ForceResolutionFrame=World  EnableTorqueX=off  EnableTorqueY=off  EnableTorqueZ=off  EnableTorque=off  TorqueResolutionFrame=AttachedFrame
  PS Constant2 : fl_lib/Physical Signals/Sources/PS Constant  constant=F_load_y
      settings: AttributesFormatString=%<constant>
  PS Constant3 : fl_lib/Physical Signals/Sources/PS Constant  constant=F_load_x
      settings: AttributesFormatString=%<constant>
  PS Math Function3 : fl_lib/Physical Signals/Functions/PS Math Function  fcn_choice=foundation.enum.math_function.reciprocal  v=1
  PS Math Function4 : fl_lib/Physical Signals/Functions/PS Math Function  fcn_choice=foundation.enum.math_function.reciprocal  v=1
  PS Product2 : fl_lib/Physical Signals/Functions/PS Product
  PS Product3 : fl_lib/Physical Signals/Functions/PS Product
  Scope : Scope
  Simulink-PS Converter2 : nesl_utility/Simulink-PS Converter  PhysicalDomain=network_engine_domain  SubClassName=ps_input  LeftPortType=input  RightPortType=output  PseudoPeriodic=off  Frequencies=[]  NoiseDistribution=none  NoiseParameters=[]  Unit=1  AffineConversion=off  FilteringAndDerivatives=provide  SimscapeFilterOrder=1  InputFilterTimeConstant=0.001  UdotUserProvided=0
  Simulink-PS Converter3 : nesl_utility/Simulink-PS Converter  PhysicalDomain=network_engine_domain  SubClassName=ps_input  LeftPortType=input  RightPortType=output  PseudoPeriodic=off  Frequencies=[]  NoiseDistribution=none  NoiseParameters=[]  Unit=1  AffineConversion=off  FilteringAndDerivatives=provide  SimscapeFilterOrder=1  InputFilterTimeConstant=0.001  UdotUserProvided=0
  To Workspace : ToWorkspace  VariableName=con_out  SampleTime=-1
  To Workspace1 : ToWorkspace  VariableName=F_load_m_out  SampleTime=-1
      settings: Decimation=3
  To Workspace2 : ToWorkspace  VariableName=t_out  SampleTime=-1
      settings: Decimation=3
  To Workspace3 : ToWorkspace  VariableName=F_load_out  SampleTime=-1
      settings: Decimation=3
  difference : Scope  NumInputPorts=2
  F : PMIOPort  Side=Right
  tag scope: con=global
  wires:
  [F_load_m] -> To Workspace1/1, difference/1, Display8/1  "F_load_measured"
  Constant/1 -> To Workspace3/1, Display12/1, difference/2  "F_load"
  Clock/1 -> To Workspace2/1
  con/1 -> To Workspace/1, [con], Scope/1, Simulink-PS Converter3/1, Simulink-PS Converter2/1  "con"
  connections:
  PS Math Function4/RConn1 -- PS Product3/LConn1
  Simulink-PS Converter2/RConn1 -- PS Math Function4/LConn1
  Simulink-PS Converter3/RConn1 -- PS Math Function3/LConn1
  PS Product2/LConn2 -- PS Constant3/RConn1
  PS Math Function3/RConn1 -- PS Product2/LConn1
  PS Constant2/RConn1 -- PS Product3/LConn2
  PS Product2/RConn1 -- External Force and Torque2/LConn1
  PS Product3/RConn1 -- External Force and Torque2/LConn2
  External Force and Torque2/RConn1 -- F/RConn1
